simulink model "mrefrobotarm_previous_y_previous_u_previous_ref_cex_3"  (R2018b)
settings: Solver=FixedStepAuto  StartTime=0.0  StopTime=20  RelTol=1e-3  AbsTol=1e-6
undefined symbols (not defined in the file or in its folder): cc, options
libraries: neural x396, simulink x2
(part 5 of 15)

== system mrefrobotarm_previous_y_previous_u_previous_ref_cex_3/cex_m1/Layer 3/Delays 1 ==
  "p{3}" : Inport  PortDimensions=30
      mask Display: e = 0.06;c1 = [120 230 180]/255;c2 = ([120 230 180]+0)/(256+128);c3 = ([120 230 180]+128)/(256+128);patch([0 1 1 0],[0 0 1 1],c1);patch([0 1 1 1-e 1-e 0+e],[0 0 1 1-e 0+e 0+e],c2);patch([0 0 1 1-e 0+e 0+e],[0 1 1 1-e 1-e 0+e],c3);plot([0 1 1 0 0],[0 0 1 1 0]);
  mux : Mux  Inputs=1
      mask Display: e = 0.06;c1 = [120 150 230]/255;c2 = ([120 150 230]+0)/383;c3 = ([120 150 230]+128)/383;patch([0 1 1 0],[0 0 1 1],c1);patch([0 1 1 1-e 1-e 0+e],[0 0 1 1-e 0+e 0+e],c2);patch([0 0 1 1-e 0+e 0+e],[0 1 1 1-e 1-e 0+e],c3);plot([0 1 1 0 0],[0 0 1 1 0]);disp('Mux')
  "pd{3,2}" : Outport
      mask Display: e = 0.06;c1 = [120 230 180]/255;c2 = ([120 230 180]+0)/(256+128);c3 = ([120 230 180]+128)/(256+128);patch([0 1 1 0],[0 0 1 1],c1);patch([0 1 1 1-e 1-e 0+e],[0 0 1 1-e 0+e 0+e],c2);patch([0 0 1 1-e 0+e 0+e],[0 1 1 1-e 1-e 0+e],c3);plot([0 1 1 0 0],[0 0 1 1 0]);
  wires:
  "p{3}"/1 -> mux/1
  mux/1 -> "pd{3,2}"/1

== system mrefrobotarm_previous_y_previous_u_previous_ref_cex_3/cex_m1/Layer 3/LW{3,2} ==
  "ad{3,2}" : Inport  PortDimensions=30
      mask Display: e = 0.06;c1 = [120 230 180]/255;c2 = ([120 230 180]+0)/(256+128);c3 = ([120 230 180]+128)/(256+128);patch([0 1 1 0],[0 0 1 1],c1);patch([0 1 1 1-e 1-e 0+e],[0 0 1 1-e 0+e 0+e],c2);patch([0 0 1 1-e 0+e 0+e],[0 1 1 1-e 1-e 0+e],c3);plot([0 1 1 0 0],[0 0 1 1 0]);
  "IW{3,2}(1,:)'" : Constant  Value=[0.0255900601227965381057050109347983379848301410675048828125;-0.2445332719523497233549136353758512996137142181396484375;0.2132234013283009488315400403735111467540264129638671875;-0.0515001036072283702171858976726070977747440338134765625;-0.19351367720373280345569355631596408784389495849609375;0.376109267327173701911391390240169130265712738037109375;0.0666749128615344577308832185735809616744518280029296875;-0.44077680308893107952172840668936260044574737548828125;-0.1774770708842355604328844265182851813733577728271484375;-0.054251675677824177934649441112924250774085521697998046875;0.407756480058180159620206950421561487019062042236328125;-0.11043832971419904886989371561867301352322101593017578125;-0.06656652324338363513334115850739181041717529296875;-0.309772314576237606242870015194057486951351165771484375;-0.2782579958208721837564780798857100307941436767578125;0.0014079282704737897634339471863995640887878835201263427734375;0.164750395979450681149813817683025263249874114990234375;0.03374371873575258973243506943617830984294414520263671875;-0.11697430223199604959471997744913096539676189422607421875;-0.377976875689660485324594674239051528275012969970703125;0.180234815360957700836053163584438152611255645751953125;0.049494338029175431736828016937579377554357051849365234375;-0.541724329864333054018743496271781623363494873046875;0.70957921545389057715880198884406127035617828369140625;-0.2236538006543592749242321815472678281366825103759765625;-0.0168625825253284934712727505257134907878935337066650390625;-0.061157151815638820246956441906149848364293575286865234375;0.0962999458349639014809184800469665788114070892333984375;-0.195422183072548050208894210300059057772159576416015625;0.469008564925858462135721538288635201752185821533203125]
      mask Display: e = 0.06;c1 = [120 150 230]/255;c2 = ([120 150 230]+0)/383;c3 = ([120 150 230]+128)/383;patch([0 1 1 0],[0 0 1 1],c1);patch([0 1 1 1-e 1-e 0+e],[0 0 1 1-e 0+e 0+e],c2);patch([0 0 1 1-e 0+e 0+e],[0 1 1 1-e 1-e 0+e],c3);plot([0 1 1 0 0],[0 0 1 1 0]);disp('weights');
  Mux : Mux  Inputs=1
      mask Display: e = 0.06;c1 = [120 150 230]/255;c2 = ([120 150 230]+0)/383;c3 = ([120 150 230]+128)/383;patch([0 1 1 0],[0 0 1 1],c1);patch([0 1 1 1-e 1-e 0+e],[0 0 1 1-e 0+e 0+e],c2);patch([0 0 1 1-e 0+e 0+e],[0 1 1 1-e 1-e 0+e],c3);plot([0 1 1 0 0],[0 0 1 1 0]);disp('Mux');
  dotprod1 : neural/Weight Functions/dotprod
  "lz{3,2}" : Outport
      mask Display: e = 0.06;c1 = [120 230 180]/255;c2 = ([120 230 180]+0)/(256+128);c3 = ([120 230 180]+128)/(256+128);patch([0 1 1 0],[0 0 1 1],c1);patch([0 1 1 1-e 1-e 0+e],[0 0 1 1-e 0+e 0+e],c2);patch([0 0 1 1-e 0+e 0+e],[0 1 1 1-e 1-e 0+e],c3);plot([0 1 1 0 0],[0 0 1 1 0]);
  wires:
  "IW{3,2}(1,:)'"/1 -> dotprod1/1
  "ad{3,2}"/1 -> dotprod1/2
  dotprod1/1 -> Mux/1
  Mux/1 -> "lz{3,2}"/1

== system mrefrobotarm_previous_y_previous_u_previous_ref_cex_3/cex_m2_adapt/Layer 1/Delays 1 ==
  "p{1}" : Inport  PortDimensions=10
      mask Display: e = 0.06;c1 = [120 230 180]/255;c2 = ([120 230 180]+0)/(256+128);c3 = ([120 230 180]+128)/(256+128);patch([0 1 1 0],[0 0 1 1],c1);patch([0 1 1 1-e 1-e 0+e],[0 0 1 1-e 0+e 0+e],c2);patch([0 0 1 1-e 0+e 0+e],[0 1 1 1-e 1-e 0+e],c3);plot([0 1 1 0 0],[0 0 1 1 0]);
  mux : Mux  Inputs=1
      mask Display: e = 0.06;c1 = [120 150 230]/255;c2 = ([120 150 230]+0)/383;c3 = ([120 150 230]+128)/383;patch([0 1 1 0],[0 0 1 1],c1);patch([0 1 1 1-e 1-e 0+e],[0 0 1 1-e 0+e 0+e],c2);patch([0 0 1 1-e 0+e 0+e],[0 1 1 1-e 1-e 0+e],c3);plot([0 1 1 0 0],[0 0 1 1 0]);disp('Mux')
  "pd{1,1}" : Outport
      mask Display: e = 0.06;c1 = [120 230 180]/255;c2 = ([120 230 180]+0)/(256+128);c3 = ([120 230 180]+128)/(256+128);patch([0 1 1 0],[0 0 1 1],c1);patch([0 1 1 1-e 1-e 0+e],[0 0 1 1-e 0+e 0+e],c2);patch([0 0 1 1-e 0+e 0+e],[0 1 1 1-e 1-e 0+e],c3);plot([0 1 1 0 0],[0 0 1 1 0]);
  wires:
  "p{1}"/1 -> mux/1
  mux/1 -> "pd{1,1}"/1

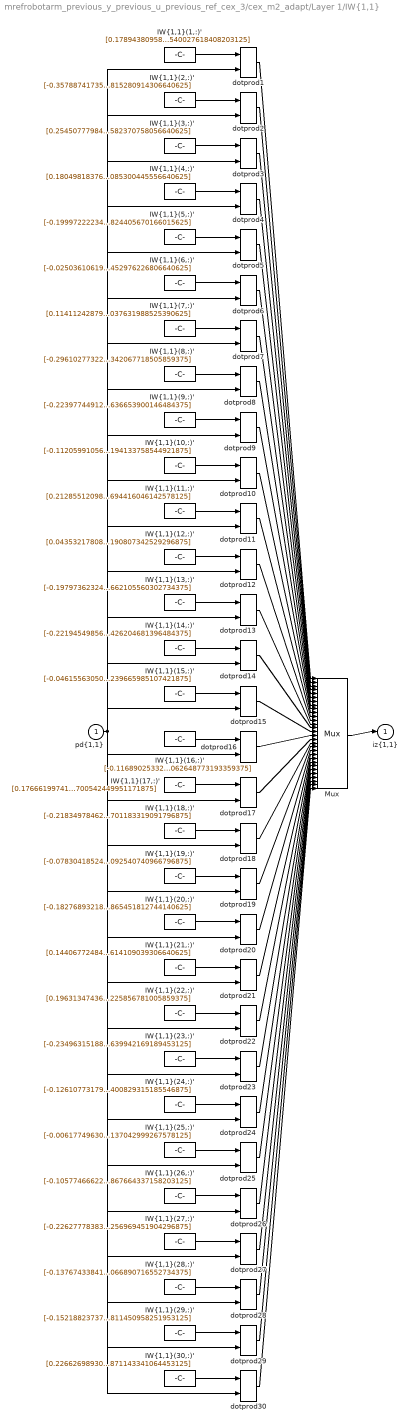
== system mrefrobotarm_previous_y_previous_u_previous_ref_cex_3/cex_m2_adapt/Layer 1/IW{1,1} ==
  "pd{1,1}" : Inport  PortDimensions=10
      mask Display: e = 0.06;c1 = [120 230 180]/255;c2 = ([120 230 180]+0)/(256+128);c3 = ([120 230 180]+128)/(256+128);patch([0 1 1 0],[0 0 1 1],c1);patch([0 1 1 1-e 1-e 0+e],[0 0 1 1-e 0+e 0+e],c2);patch([0 0 1 1-e 0+e 0+e],[0 1 1 1-e 1-e 0+e],c3);plot([0 1 1 0 0],[0 0 1 1 0]);
  "IW{1,1}(1,:)'" : Constant  Value=[0.17894380958113875745851828469312749803066253662109375;0.0268071317300851152953811151746776886284351348876953125;-0.0194245512122687945255616881468085921369493007659912109375;-0.08160327981400332386652252125713857822120189666748046875;-0.09141169433945516009654141953433281742036342620849609375;-0.0300313493066236281148206899160868488252162933349609375;-0.282419827211167984160056221298873424530029296875;0.1311114560309999121923141274237423203885555267333984375;-0.18958968204741710739114068928756751120090484619140625;0.2425038701812252117662183081847615540027618408203125]
      mask Display: e = 0.06;c1 = [120 150 230]/255;c2 = ([120 150 230]+0)/383;c3 = ([120 150 230]+128)/383;patch([0 1 1 0],[0 0 1 1],c1);patch([0 1 1 1-e 1-e 0+e],[0 0 1 1-e 0+e 0+e],c2);patch([0 0 1 1-e 0+e 0+e],[0 1 1 1-e 1-e 0+e],c3);plot([0 1 1 0 0],[0 0 1 1 0]);disp('Weights');
  "IW{1,1}(10,:)'" : Constant  Value=[-0.11205991056579979459062457181062200106680393218994140625;0.357141388765579048669707162844133563339710235595703125;-0.24716782224828592884335876078694127500057220458984375;0.0269643266049996131739074911592979333363473415374755859375;0.33336725590618654369023943218053318560123443603515625;-0.3923495977236670650967198525904677808284759521484375;0.1045060443543400496846373926018713973462581634521484375;-0.06697855843020487920380645618934067897498607635498046875;-0.0864082527450108772715253735441365279257297515869140625;-0.39109248089432480099958411301486194133758544921875]
      mask Display: e = 0.06;c1 = [120 150 230]/255;c2 = ([120 150 230]+0)/383;c3 = ([120 150 230]+128)/383;patch([0 1 1 0],[0 0 1 1],c1);patch([0 1 1 1-e 1-e 0+e],[0 0 1 1-e 0+e 0+e],c2);patch([0 0 1 1-e 0+e 0+e],[0 1 1 1-e 1-e 0+e],c3);plot([0 1 1 0 0],[0 0 1 1 0]);disp('Weights');
  "IW{1,1}(11,:)'" : Constant  Value=[0.2128551209829567525400051408723811618983745574951171875;-0.2022275282815631236577047502578352577984333038330078125;0.0248801394003134446197833540281862951815128326416015625;-0.152377187466551433647765634304960258305072784423828125;0.01342328889111928623412151040383832878433167934417724609375;0.33377738714321558699538172731990925967693328857421875;-0.12204906903726205069649068946091574616730213165283203125;0.154449232987741658096325636506662704050540924072265625;-0.029966565392852896609898749602507450617849826812744140625;0.1513983111497898825792418620039825327694416046142578125]
      mask Display: e = 0.06;c1 = [120 150 230]/255;c2 = ([120 150 230]+0)/383;c3 = ([120 150 230]+128)/383;patch([0 1 1 0],[0 0 1 1],c1);patch([0 1 1 1-e 1-e 0+e],[0 0 1 1-e 0+e 0+e],c2);patch([0 0 1 1-e 0+e 0+e],[0 1 1 1-e 1-e 0+e],c3);plot([0 1 1 0 0],[0 0 1 1 0]);disp('Weights');
  "IW{1,1}(12,:)'" : Constant  Value=[0.043532178080436627343186017924381303600966930389404296875;-0.41453145188763296236089672675007022917270660400390625;0.215272607105115143522056087022065185010433197021484375;0.1665664633557482066095190020860172808170318603515625;-0.02357860495869094907828156237883376888930797576904296875;0.0857323194401150845411763157244422473013401031494140625;-0.1958108534085869489871356563526205718517303466796875;-0.1625029873389834123020847300722380168735980987548828125;0.25121695445630820575644293057848699390888214111328125;-0.106927667380184832079947909733164124190807342529296875]
      mask Display: e = 0.06;c1 = [120 150 230]/255;c2 = ([120 150 230]+0)/383;c3 = ([120 150 230]+128)/383;patch([0 1 1 0],[0 0 1 1],c1);patch([0 1 1 1-e 1-e 0+e],[0 0 1 1-e 0+e 0+e],c2);patch([0 0 1 1-e 0+e 0+e],[0 1 1 1-e 1-e 0+e],c3);plot([0 1 1 0 0],[0 0 1 1 0]);disp('Weights');
  "IW{1,1}(13,:)'" : Constant  Value=[-0.197973623241752105794688532114378176629543304443359375;0.1845413812524343832865980630231206305325031280517578125;-0.06383679347059974251710201542664435692131519317626953125;0.2121214746879949430979905855565448291599750518798828125;-0.1380893753585880900924820480213384144008159637451171875;0.038970623662596674818825448483039508573710918426513671875;0.1056184031157495761821252244772040285170078277587890625;-0.1502218965172570086519243659495259635150432586669921875;-0.246327164138165410900427332308026961982250213623046875;0.2171770133514413225750416813752963207662105560302734375]
      mask Display: e = 0.06;c1 = [120 150 230]/255;c2 = ([120 150 230]+0)/383;c3 = ([120 150 230]+128)/383;patch([0 1 1 0],[0 0 1 1],c1);patch([0 1 1 1-e 1-e 0+e],[0 0 1 1-e 0+e 0+e],c2);patch([0 0 1 1-e 0+e 0+e],[0 1 1 1-e 1-e 0+e],c3);plot([0 1 1 0 0],[0 0 1 1 0]);disp('Weights');
  "IW{1,1}(14,:)'" : Constant  Value=[-0.2219454985619064846247283639968372881412506103515625;-0.031461568819169304089822247760821483097970485687255859375;0.25100732039812767570907681147218681871891021728515625;-0.071675964588810925359751990981749258935451507568359375;-0.017276940888944262997295453487822669558227062225341796875;0.18731594061744616386278039499302394688129425048828125;0.190073867922183448175843523131334222853183746337890625;0.25628758967802023338578010225319303572177886962890625;-0.12311552773296086105148106071283109486103057861328125;0.0836877380832282413702927215126692317426204681396484375]
      mask Display: e = 0.06;c1 = [120 150 230]/255;c2 = ([120 150 230]+0)/383;c3 = ([120 150 230]+128)/383;patch([0 1 1 0],[0 0 1 1],c1);patch([0 1 1 1-e 1-e 0+e],[0 0 1 1-e 0+e 0+e],c2);patch([0 0 1 1-e 0+e 0+e],[0 1 1 1-e 1-e 0+e],c3);plot([0 1 1 0 0],[0 0 1 1 0]);disp('Weights');
  "IW{1,1}(15,:)'" : Constant  Value=[-0.0461556305026336877173065431634313426911830902099609375;-0.150134721130089798801776623804471455514430999755859375;0.009230602670664188325044818839160143397748470306396484375;-0.263036107154839104982357866902020759880542755126953125;-0.23279760428147711071034109409083612263202667236328125;-0.2026113135926179975587757553512346930801868438720703125;0.051737200499545492327069240445780451409518718719482421875;-0.209756927138399051901984648793586529791355133056640625;0.18107018174338918026222700063954107463359832763671875;-0.037977675462847075571470867316747899167239665985107421875]
      mask Display: e = 0.06;c1 = [120 150 230]/255;c2 = ([120 150 230]+0)/383;c3 = ([120 150 230]+128)/383;patch([0 1 1 0],[0 0 1 1],c1);patch([0 1 1 1-e 1-e 0+e],[0 0 1 1-e 0+e 0+e],c2);patch([0 0 1 1-e 0+e 0+e],[0 1 1 1-e 1-e 0+e],c3);plot([0 1 1 0 0],[0 0 1 1 0]);disp('Weights');
  "IW{1,1}(16,:)'" : Constant  Value=[-0.116890253323373605187640578151331283152103424072265625;0.1948278121702989029717656421780702657997608184814453125;0.2451443399859792038331107733029057271778583526611328125;0.0631447386421812861811986294924281537532806396484375;-0.17107126514984816179065774122136645019054412841796875;0.2286361380735318082901841307830181904137134552001953125;0.1679551899195639574902116919474792666733264923095703125;-0.1360221986945425454162972300764522515237331390380859375;0.1710850103284725365337948232991038821637630462646484375;-0.03517712954871109187759969927355996333062648773193359375]
      mask Display: e = 0.06;c1 = [120 150 230]/255;c2 = ([120 150 230]+0)/383;c3 = ([120 150 230]+128)/383;patch([0 1 1 0],[0 0 1 1],c1);patch([0 1 1 1-e 1-e 0+e],[0 0 1 1-e 0+e 0+e],c2);patch([0 0 1 1-e 0+e 0+e],[0 1 1 1-e 1-e 0+e],c3);plot([0 1 1 0 0],[0 0 1 1 0]);disp('Weights');
  "IW{1,1}(17,:)'" : Constant  Value=[0.1766619974178879892701132803267682902514934539794921875;-0.0792409472181059559847682294275728054344654083251953125;-0.0793088341233295912591216847431496717035770416259765625;-0.1959233532531541588372903106574085541069507598876953125;0.11565209295813162759802850132473395206034183502197265625;0.00787878799489242533093946718736333423294126987457275390625;0.042692546684134226320228577833404415287077426910400390625;-0.209397876134871430142680992503301240503787994384765625;-0.17372430623133772176203137860284186899662017822265625;-0.30776366573309743568387375489692203700542449951171875]
      mask Display: e = 0.06;c1 = [120 150 230]/255;c2 = ([120 150 230]+0)/383;c3 = ([120 150 230]+128)/383;patch([0 1 1 0],[0 0 1 1],c1);patch([0 1 1 1-e 1-e 0+e],[0 0 1 1-e 0+e 0+e],c2);patch([0 0 1 1-e 0+e 0+e],[0 1 1 1-e 1-e 0+e],c3);plot([0 1 1 0 0],[0 0 1 1 0]);disp('Weights');
  "IW{1,1}(18,:)'" : Constant  Value=[-0.218349784629069620933705664356239140033721923828125;0.0642278208810374284798427879650262184441089630126953125;-0.0619524210695374388802036946799489669501781463623046875;0.09804765153544270361862800200469791889190673828125;-0.1940721708608581508315182873047888278961181640625;0.10055382144939296884533774800729588605463504791259765625;0.055125079744373917112199023904395289719104766845703125;-0.22257044783044499514090830416535027325153350830078125;0.307695206730231929359575815396965481340885162353515625;0.035102723566185704828779279296213644556701183319091796875]
      mask Display: e = 0.06;c1 = [120 150 230]/255;c2 = ([120 150 230]+0)/383;c3 = ([120 150 230]+128)/383;patch([0 1 1 0],[0 0 1 1],c1);patch([0 1 1 1-e 1-e 0+e],[0 0 1 1-e 0+e 0+e],c2);patch([0 0 1 1-e 0+e 0+e],[0 1 1 1-e 1-e 0+e],c3);plot([0 1 1 0 0],[0 0 1 1 0]);disp('Weights');
  "IW{1,1}(19,:)'" : Constant  Value=[-0.0783041852438026986238384097305242903530597686767578125;-0.110159278051770892492555731223546899855136871337890625;0.0703702840684951869132390811500954441726207733154296875;-0.07371581746469789420128648771424195729196071624755859375;0.249837105675603743382140464746044017374515533447265625;-0.1447885961919746222736904428529669530689716339111328125;0.321300374598912752421853156192810274660587310791015625;0.0142112607252117585654449527510223560966551303863525390625;-0.2097588763900186392685753844489227049052715301513671875;-0.137897701114751913831213414596277289092540740966796875]
      mask Display: e = 0.06;c1 = [120 150 230]/255;c2 = ([120 150 230]+0)/383;c3 = ([120 150 230]+128)/383;patch([0 1 1 0],[0 0 1 1],c1);patch([0 1 1 1-e 1-e 0+e],[0 0 1 1-e 0+e 0+e],c2);patch([0 0 1 1-e 0+e 0+e],[0 1 1 1-e 1-e 0+e],c3);plot([0 1 1 0 0],[0 0 1 1 0]);disp('Weights');
  "IW{1,1}(2,:)'" : Constant  Value=[-0.3578874173535078195840242187841795384883880615234375;-0.170151089097431207353139370752614922821521759033203125;0.1283993877341979839012964248468051664531230926513671875;0.0278821277396804866055557425852384767495095729827880859375;0.241336606408127651857142836888669990003108978271484375;-0.088299581297500984167214710396365262567996978759765625;-0.05964540699157604153324285789494751952588558197021484375;-0.18177101439334253374369154698797501623630523681640625;-0.202751370739727987402289954843581654131412506103515625;0.03612164991689260917784309867784031666815280914306640625]
      mask Display: e = 0.06;c1 = [120 150 230]/255;c2 = ([120 150 230]+0)/383;c3 = ([120 150 230]+128)/383;patch([0 1 1 0],[0 0 1 1],c1);patch([0 1 1 1-e 1-e 0+e],[0 0 1 1-e 0+e 0+e],c2);patch([0 0 1 1-e 0+e 0+e],[0 1 1 1-e 1-e 0+e],c3);plot([0 1 1 0 0],[0 0 1 1 0]);disp('Weights');
  "IW{1,1}(20,:)'" : Constant  Value=[-0.182768932186715804544263619391131214797496795654296875;0.429775783628007890246891520291683264076709747314453125;0.047518314508741339718955742910111439414322376251220703125;-0.051709077215492692258802520655081025324761867523193359375;0.091944243252948643085886715198284946382045745849609375;-0.378830904703480075834676199519890360534191131591796875;-0.03264809407481177039311859289227868430316448211669921875;-0.035928795977489068336208077880655764602124691009521484375;-0.0821954152999051779193706579462741501629352569580078125;-0.122911018759520873633306337069370783865451812744140625]
      mask Display: e = 0.06;c1 = [120 150 230]/255;c2 = ([120 150 230]+0)/383;c3 = ([120 150 230]+128)/383;patch([0 1 1 0],[0 0 1 1],c1);patch([0 1 1 1-e 1-e 0+e],[0 0 1 1-e 0+e 0+e],c2);patch([0 0 1 1-e 0+e 0+e],[0 1 1 1-e 1-e 0+e],c3);plot([0 1 1 0 0],[0 0 1 1 0]);disp('Weights');
  "IW{1,1}(21,:)'" : Constant  Value=[0.1440677248405341226433762358283274807035923004150390625;0.05674263640774103445441056692288839258253574371337890625;0.186993057845454779819505120030953548848628997802734375;-0.1647920441410975767038138428688398562371730804443359375;-0.23737996741754530116708110654144547879695892333984375;0.253688660892035511285058646535617299377918243408203125;-0.2346548398854706451999163618893362581729888916015625;0.0215902337998425848664130199949795496650040149688720703125;0.2383889116336310731725234290934167802333831787109375;-0.0025995181104539661666452676769267782219685614109039306640625]
      mask Display: e = 0.06;c1 = [120 150 230]/255;c2 = ([120 150 230]+0)/383;c3 = ([120 150 230]+128)/383;patch([0 1 1 0],[0 0 1 1],c1);patch([0 1 1 1-e 1-e 0+e],[0 0 1 1-e 0+e 0+e],c2);patch([0 0 1 1-e 0+e 0+e],[0 1 1 1-e 1-e 0+e],c3);plot([0 1 1 0 0],[0 0 1 1 0]);disp('Weights');
  "IW{1,1}(22,:)'" : Constant  Value=[0.1963134743628309752949689936940558254718780517578125;-0.05200275022295146321038572523320908658206462860107421875;-0.2715367927651737289806987973861396312713623046875;-0.08952620051789726696167548425364657305181026458740234375;-0.036953019016694517440146938724865322001278400421142578125;0.004476533827437712519115020626259138225577771663665771484375;0.259201846168678973203469695363310165703296661376953125;-0.08894573404800827642890936886033159680664539337158203125;0.032269069594959988445115328659085207618772983551025390625;0.306951271732894992450013660345575772225856781005859375]
      mask Display: e = 0.06;c1 = [120 150 230]/255;c2 = ([120 150 230]+0)/383;c3 = ([120 150 230]+128)/383;patch([0 1 1 0],[0 0 1 1],c1);patch([0 1 1 1-e 1-e 0+e],[0 0 1 1-e 0+e 0+e],c2);patch([0 0 1 1-e 0+e 0+e],[0 1 1 1-e 1-e 0+e],c3);plot([0 1 1 0 0],[0 0 1 1 0]);disp('Weights');
  "IW{1,1}(23,:)'" : Constant  Value=[-0.2349631518819057240943237729879911057651042938232421875;-0.17641433096250180856401357232243753969669342041015625;0.23491215286060407319013165761134587228298187255859375;0.0979759738956398062992292352646472863852977752685546875;0.275412544487549648675184243984404020011425018310546875;-0.006673035133562527261574803816301937331445515155792236328125;-0.086308845438423376084102756067295558750629425048828125;-0.04925444461655315020465195630094967782497406005859375;0.311981159375483707574261416084482334554195404052734375;-0.13017093754148068018849926374969072639942169189453125]
      mask Display: e = 0.06;c1 = [120 150 230]/255;c2 = ([120 150 230]+0)/383;c3 = ([120 150 230]+128)/383;patch([0 1 1 0],[0 0 1 1],c1);patch([0 1 1 1-e 1-e 0+e],[0 0 1 1-e 0+e 0+e],c2);patch([0 0 1 1-e 0+e 0+e],[0 1 1 1-e 1-e 0+e],c3);plot([0 1 1 0 0],[0 0 1 1 0]);disp('Weights');
  "IW{1,1}(24,:)'" : Constant  Value=[-0.126107731797233502124555570844677276909351348876953125;0.0845353935998513772442919389504822902381420135498046875;-0.170961691516502922727482882692129351198673248291015625;0.2911848648253305693600623271777294576168060302734375;0.1152242375241279426223428572484408505260944366455078125;0.270250526997318607502762688454822637140750885009765625;0.11501804092393873302224704957552603445947170257568359375;0.06893195638638706379541787327980273403227329254150390625;0.09231210104422175877214584716057288460433483123779296875;0.12574616199281507533669355325400829315185546875]
      mask Display: e = 0.06;c1 = [120 150 230]/255;c2 = ([120 150 230]+0)/383;c3 = ([120 150 230]+128)/383;patch([0 1 1 0],[0 0 1 1],c1);patch([0 1 1 1-e 1-e 0+e],[0 0 1 1-e 0+e 0+e],c2);patch([0 0 1 1-e 0+e 0+e],[0 1 1 1-e 1-e 0+e],c3);plot([0 1 1 0 0],[0 0 1 1 0]);disp('Weights');
  "IW{1,1}(25,:)'" : Constant  Value=[-0.0061774963028770855932858552250763750635087490081787109375;0.1585491037024161775637054461185471154749393463134765625;0.188599532141205228352731637642136774957180023193359375;-0.01688017055565992075027992314062430523335933685302734375;-0.18879192571435854386407982019591145217418670654296875;0.1272448344067560188630494621975230984389781951904296875;-0.018569046672616905391262065450064255855977535247802734375;0.2719719856826794401882807505899108946323394775390625;0.11406227701772338190000510849131387658417224884033203125;-0.2380939274560498752908443975684349425137042999267578125]
      mask Display: e = 0.06;c1 = [120 150 230]/255;c2 = ([120 150 230]+0)/383;c3 = ([120 150 230]+128)/383;patch([0 1 1 0],[0 0 1 1],c1);patch([0 1 1 1-e 1-e 0+e],[0 0 1 1-e 0+e 0+e],c2);patch([0 0 1 1-e 0+e 0+e],[0 1 1 1-e 1-e 0+e],c3);plot([0 1 1 0 0],[0 0 1 1 0]);disp('Weights');
  "IW{1,1}(26,:)'" : Constant  Value=[-0.10577466622952902408627551267272792756557464599609375;0.178203524722881312403188758253236301243305206298828125;-0.257770785536782287561408111287164501845836639404296875;-0.12118946165142341353515575974597595632076263427734375;0.1079912289210649134485464628596673719584941864013671875;0.03241305524148041516951934681856073439121246337890625;0.23392595501652213574317329403129406273365020751953125;0.04862524796426924422743098830324015580117702484130859375;-0.07777126056271836673783326432385365478694438934326171875;-0.066068618504620257869675015172106213867664337158203125]
      mask Display: e = 0.06;c1 = [120 150 230]/255;c2 = ([120 150 230]+0)/383;c3 = ([120 150 230]+128)/383;patch([0 1 1 0],[0 0 1 1],c1);patch([0 1 1 1-e 1-e 0+e],[0 0 1 1-e 0+e 0+e],c2);patch([0 0 1 1-e 0+e 0+e],[0 1 1 1-e 1-e 0+e],c3);plot([0 1 1 0 0],[0 0 1 1 0]);disp('Weights');
  "IW{1,1}(27,:)'" : Constant  Value=[-0.22627778383142194140731362494989298284053802490234375;0.2283804303486903497510951410731649957597255706787109375;-0.04633207616607355749938079725325223989784717559814453125;-0.2155678259000181895554959510263870470225811004638671875;-0.024473322781653643331889469436646322719752788543701171875;-0.061312110441402466187721387314013554714620113372802734375;0.192636598116036783512328156575676985085010528564453125;0.2137994347702246444864471186519949696958065032958984375;0.240218978868222909905938422525650821626186370849609375;0.00468413039874411400720344289538843440823256969451904296875]
      mask Display: e = 0.06;c1 = [120 150 230]/255;c2 = ([120 150 230]+0)/383;c3 = ([120 150 230]+128)/383;patch([0 1 1 0],[0 0 1 1],c1);patch([0 1 1 1-e 1-e 0+e],[0 0 1 1-e 0+e 0+e],c2);patch([0 0 1 1-e 0+e 0+e],[0 1 1 1-e 1-e 0+e],c3);plot([0 1 1 0 0],[0 0 1 1 0]);disp('Weights');
  "IW{1,1}(28,:)'" : Constant  Value=[-0.1376743384100590217311577134751132689416408538818359375;0.135728354626229730239828086268971674144268035888671875;0.109024380491910488633067188857239671051502227783203125;-0.020932506514744549097617465349685517139732837677001953125;0.1596172013299924363760595724670565687119960784912109375;-0.2246346884976990754267944794264622032642364501953125;-0.126744927810719054672716765708173625171184539794921875;0.152022505625554471553328994559706188738346099853515625;0.2181400746204700258346065311343409121036529541015625;-0.047226325411993307079594472952521755360066890716552734375]
      mask Display: e = 0.06;c1 = [120 150 230]/255;c2 = ([120 150 230]+0)/383;c3 = ([120 150 230]+128)/383;patch([0 1 1 0],[0 0 1 1],c1);patch([0 1 1 1-e 1-e 0+e],[0 0 1 1-e 0+e 0+e],c2);patch([0 0 1 1-e 0+e 0+e],[0 1 1 1-e 1-e 0+e],c3);plot([0 1 1 0 0],[0 0 1 1 0]);disp('Weights');
  "IW{1,1}(29,:)'" : Constant  Value=[-0.1521882373734292637212917043143534101545810699462890625;-0.0458248690782084022732334460670244880020618438720703125;0.07555221417059405919491865688542020507156848907470703125;-0.1852621927616607544475613167378469370305538177490234375;0.15125110154184862043535986231290735304355621337890625;-0.1412090535903816890250794813255197368562221527099609375;-0.08681811528340076244969480967483832500874996185302734375;-0.224873363801992687260877801236347295343875885009765625;-0.165199621824701325945028429487138055264949798583984375;0.157553748575570029544223871198482811450958251953125]
      mask Display: e = 0.06;c1 = [120 150 230]/255;c2 = ([120 150 230]+0)/383;c3 = ([120 150 230]+128)/383;patch([0 1 1 0],[0 0 1 1],c1);patch([0 1 1 1-e 1-e 0+e],[0 0 1 1-e 0+e 0+e],c2);patch([0 0 1 1-e 0+e 0+e],[0 1 1 1-e 1-e 0+e],c3);plot([0 1 1 0 0],[0 0 1 1 0]);disp('Weights');
  "IW{1,1}(3,:)'" : Constant  Value=[0.2545077798497317189685418270528316497802734375;0.040200776831324842863768509459987399168312549591064453125;0.16885528047504616555585243986570276319980621337890625;0.227543951883704076433190266470774076879024505615234375;0.2384163836713796558175459949779906310141086578369140625;0.1413290689938786204304932425657170824706554412841796875;0.10575857589675634329307030156996916048228740692138671875;0.133407682047404663183698403372545726597309112548828125;0.12030518109430683726390753918167320080101490020751953125;0.11598616257945094931702811891227611340582370758056640625]
      mask Display: e = 0.06;c1 = [120 150 230]/255;c2 = ([120 150 230]+0)/383;c3 = ([120 150 230]+128)/383;patch([0 1 1 0],[0 0 1 1],c1);patch([0 1 1 1-e 1-e 0+e],[0 0 1 1-e 0+e 0+e],c2);patch([0 0 1 1-e 0+e 0+e],[0 1 1 1-e 1-e 0+e],c3);plot([0 1 1 0 0],[0 0 1 1 0]);disp('Weights');
  "IW{1,1}(30,:)'" : Constant  Value=[0.226626989308528814515142357777222059667110443115234375;0.1400904348982205671614309494543704204261302947998046875;-0.11186941054087540248218601846019737422466278076171875;0.2012528084778613945982073119012056849896907806396484375;-0.018626897424557094240515908722954918630421161651611328125;-0.200639757261653117748068098080693744122982025146484375;-0.0961578448371694094465311763997306115925312042236328125;-0.177214676264387749338169442125945352017879486083984375;0.031918329000240552861811238472000695765018463134765625;0.266965554029287677195725336787290871143341064453125]
      mask Display: e = 0.06;c1 = [120 150 230]/255;c2 = ([120 150 230]+0)/383;c3 = ([120 150 230]+128)/383;patch([0 1 1 0],[0 0 1 1],c1);patch([0 1 1 1-e 1-e 0+e],[0 0 1 1-e 0+e 0+e],c2);patch([0 0 1 1-e 0+e 0+e],[0 1 1 1-e 1-e 0+e],c3);plot([0 1 1 0 0],[0 0 1 1 0]);disp('Weights');
  "IW{1,1}(4,:)'" : Constant  Value=[0.180498183761611807884861491402261890470981597900390625;-0.2288560682142836977259747754942509345710277557373046875;0.181865366464034339255562144899158738553524017333984375;-0.03794964346253447418089166376375942490994930267333984375;-0.00539640154973875484090140020043691038154065608978271484375;0.1827887046756515310175217337018693797290325164794921875;-0.05529857869917853552266251426772214472293853759765625;-0.1474419509970783248586911895472439937293529510498046875;-0.27933067356285434801321798659046180546283721923828125;0.1322504052913414940295666610836633481085300445556640625]
      mask Display: e = 0.06;c1 = [120 150 230]/255;c2 = ([120 150 230]+0)/383;c3 = ([120 150 230]+128)/383;patch([0 1 1 0],[0 0 1 1],c1);patch([0 1 1 1-e 1-e 0+e],[0 0 1 1-e 0+e 0+e],c2);patch([0 0 1 1-e 0+e 0+e],[0 1 1 1-e 1-e 0+e],c3);plot([0 1 1 0 0],[0 0 1 1 0]);disp('Weights');
  "IW{1,1}(5,:)'" : Constant  Value=[-0.199972222347502948114339460516930557787418365478515625;-0.1629616266957280845684152836838620714843273162841796875;-0.1088061844054873106291125850475509651005268096923828125;0.0511308765597847936223985243486822582781314849853515625;-0.0237228601571770163214392113104622694663703441619873046875;0.05171937119826557072155281957748229615390300750732421875;-0.1720231930632351302623561650761985220015048980712890625;-0.2044816792317828146874347794437198899686336517333984375;0.1663037605507071692301224175025708973407745361328125;-0.1391865350676850798805617159814573824405670166015625]
      mask Display: e = 0.06;c1 = [120 150 230]/255;c2 = ([120 150 230]+0)/383;c3 = ([120 150 230]+128)/383;patch([0 1 1 0],[0 0 1 1],c1);patch([0 1 1 1-e 1-e 0+e],[0 0 1 1-e 0+e 0+e],c2);patch([0 0 1 1-e 0+e 0+e],[0 1 1 1-e 1-e 0+e],c3);plot([0 1 1 0 0],[0 0 1 1 0]);disp('Weights');
  "IW{1,1}(6,:)'" : Constant  Value=[-0.025036106197230699466071968117830692790448665618896484375;-0.004459099454261481083883200682294045691378414630889892578125;0.06640331129765809914378138500978820957243442535400390625;-0.213060680378278355373566910202498547732830047607421875;0.1292960241831762335795730223253485746681690216064453125;-0.134777908717993444298599570174701511859893798828125;-0.2359873783413052594770675796098657883703708648681640625;-0.06528979964846935712952102903727791272103786468505859375;-0.14430156278261174751520456993603147566318511962890625;0.0887677052430439206265333496048697270452976226806640625]
      mask Display: e = 0.06;c1 = [120 150 230]/255;c2 = ([120 150 230]+0)/383;c3 = ([120 150 230]+128)/383;patch([0 1 1 0],[0 0 1 1],c1);patch([0 1 1 1-e 1-e 0+e],[0 0 1 1-e 0+e 0+e],c2);patch([0 0 1 1-e 0+e 0+e],[0 1 1 1-e 1-e 0+e],c3);plot([0 1 1 0 0],[0 0 1 1 0]);disp('Weights');
  "IW{1,1}(7,:)'" : Constant  Value=[0.11411242879864545718415769215425825677812099456787109375;-0.0719764546582311870448478430262184701859951019287109375;0.2194207952041006548515866825255216099321842193603515625;0.208720306017479206861509055670467205345630645751953125;0.042791162240613418721313365722380694933235645294189453125;0.0121936122546550916589946922385934158228337764739990234375;0.10314935925821260009893620690490934066474437713623046875;0.2155964619388381631193141174662741832435131072998046875;-0.112014458972907127165541396607295610010623931884765625;0.26768961478474262438709274647408165037631988525390625]
      mask Display: e = 0.06;c1 = [120 150 230]/255;c2 = ([120 150 230]+0)/383;c3 = ([120 150 230]+128)/383;patch([0 1 1 0],[0 0 1 1],c1);patch([0 1 1 1-e 1-e 0+e],[0 0 1 1-e 0+e 0+e],c2);patch([0 0 1 1-e 0+e 0+e],[0 1 1 1-e 1-e 0+e],c3);plot([0 1 1 0 0],[0 0 1 1 0]);disp('Weights');
  "IW{1,1}(8,:)'" : Constant  Value=[-0.2961027732226113595714878101716749370098114013671875;-0.07463399570507878166836235322989523410797119140625;-0.23855500073995183907271666612359695136547088623046875;-0.2056116722217617709400627745708334259688854217529296875;0.052565443905320197170993878899025730788707733154296875;-0.1454334110053014939012427930720150470733642578125;0.1567884249944997698822390930217807181179523468017578125;0.1721666479786218284520060706199728883802890777587890625;-0.0903178064951806192084404756315052509307861328125;-0.0525141546112134205426258404258987866342067718505859375]
      mask Display: e = 0.06;c1 = [120 150 230]/255;c2 = ([120 150 230]+0)/383;c3 = ([120 150 230]+128)/383;patch([0 1 1 0],[0 0 1 1],c1);patch([0 1 1 1-e 1-e 0+e],[0 0 1 1-e 0+e 0+e],c2);patch([0 0 1 1-e 0+e 0+e],[0 1 1 1-e 1-e 0+e],c3);plot([0 1 1 0 0],[0 0 1 1 0]);disp('Weights');
  "IW{1,1}(9,:)'" : Constant  Value=[-0.2239774491285566326848055496157030574977397918701171875;-0.1882933671208217030201836905689560808241367340087890625;-0.0257943275412955246028712252837067353539168834686279296875;0.07815168279298902176410734909950406290590763092041015625;0.0356263752072844275264884572607115842401981353759765625;-0.0373208609766592369627602465698146261274814605712890625;-0.28071250177076212395377297070808708667755126953125;0.326090076060244260514053848964977078139781951904296875;0.052075518180411901891790904528534156270325183868408203125;-0.0171626285640969454548976358410072862170636653900146484375]
      mask Display: e = 0.06;c1 = [120 150 230]/255;c2 = ([120 150 230]+0)/383;c3 = ([120 150 230]+128)/383;patch([0 1 1 0],[0 0 1 1],c1);patch([0 1 1 1-e 1-e 0+e],[0 0 1 1-e 0+e 0+e],c2);patch([0 0 1 1-e 0+e 0+e],[0 1 1 1-e 1-e 0+e],c3);plot([0 1 1 0 0],[0 0 1 1 0]);disp('Weights');
  Mux : Mux  Inputs=30
      mask Display: e = 0.06;c1 = [120 150 230]/255;c2 = ([120 150 230]+0)/383;c3 = ([120 150 230]+128)/383;patch([0 1 1 0],[0 0 1 1],c1);patch([0 1 1 1-e 1-e 0+e],[0 0 1 1-e 0+e 0+e],c2);patch([0 0 1 1-e 0+e 0+e],[0 1 1 1-e 1-e 0+e],c3);plot([0 1 1 0 0],[0 0 1 1 0]);disp('Mux');
  dotprod{1..30} (30 alike) : neural/Weight Functions/dotprod
  "iz{1,1}" : Outport
      mask Display: e = 0.06;c1 = [120 230 180]/255;c2 = ([120 230 180]+0)/(256+128);c3 = ([120 230 180]+128)/(256+128);patch([0 1 1 0],[0 0 1 1],c1);patch([0 1 1 1-e 1-e 0+e],[0 0 1 1-e 0+e 0+e],c2);patch([0 0 1 1-e 0+e 0+e],[0 1 1 1-e 1-e 0+e],c3);plot([0 1 1 0 0],[0 0 1 1 0]);
  wires:
  "IW{1,1}(1,:)'"/1 -> dotprod1/1
  "pd{1,1}"/1 -> dotprod1/2, dotprod2/2, dotprod3/2, dotprod4/2, dotprod5/2, dotprod6/2, dotprod7/2, dotprod8/2, dotprod9/2, dotprod10/2, dotprod11/2, dotprod12/2, dotprod13/2, dotprod14/2, dotprod15/2, dotprod16/2, dotprod17/2, dotprod18/2, dotprod19/2, dotprod20/2, dotprod21/2, dotprod22/2, dotprod23/2, dotprod24/2, dotprod25/2, dotprod26/2, dotprod27/2, dotprod28/2, dotprod29/2, dotprod30/2
  dotprod1/1 -> Mux/1
  "IW{1,1}(2,:)'"/1 -> dotprod2/1
  dotprod2/1 -> Mux/2
  "IW{1,1}(3,:)'"/1 -> dotprod3/1
  dotprod3/1 -> Mux/3
  "IW{1,1}(4,:)'"/1 -> dotprod4/1
  dotprod4/1 -> Mux/4
  "IW{1,1}(5,:)'"/1 -> dotprod5/1
  dotprod5/1 -> Mux/5
  "IW{1,1}(6,:)'"/1 -> dotprod6/1
  dotprod6/1 -> Mux/6
  "IW{1,1}(7,:)'"/1 -> dotprod7/1
  dotprod7/1 -> Mux/7
  "IW{1,1}(8,:)'"/1 -> dotprod8/1
  dotprod8/1 -> Mux/8
  "IW{1,1}(9,:)'"/1 -> dotprod9/1
  dotprod9/1 -> Mux/9
  "IW{1,1}(10,:)'"/1 -> dotprod10/1
  dotprod10/1 -> Mux/10
  "IW{1,1}(11,:)'"/1 -> dotprod11/1
  dotprod11/1 -> Mux/11
  "IW{1,1}(12,:)'"/1 -> dotprod12/1
  dotprod12/1 -> Mux/12
  "IW{1,1}(13,:)'"/1 -> dotprod13/1
  dotprod13/1 -> Mux/13
  "IW{1,1}(14,:)'"/1 -> dotprod14/1
  dotprod14/1 -> Mux/14
  "IW{1,1}(15,:)'"/1 -> dotprod15/1
  dotprod15/1 -> Mux/15
  "IW{1,1}(16,:)'"/1 -> dotprod16/1
  dotprod16/1 -> Mux/16
  "IW{1,1}(17,:)'"/1 -> dotprod17/1
  dotprod17/1 -> Mux/17
  "IW{1,1}(18,:)'"/1 -> dotprod18/1
  dotprod18/1 -> Mux/18
  "IW{1,1}(19,:)'"/1 -> dotprod19/1
  dotprod19/1 -> Mux/19
  "IW{1,1}(20,:)'"/1 -> dotprod20/1
  dotprod20/1 -> Mux/20
  "IW{1,1}(21,:)'"/1 -> dotprod21/1
  dotprod21/1 -> Mux/21
  "IW{1,1}(22,:)'"/1 -> dotprod22/1
  dotprod22/1 -> Mux/22
  "IW{1,1}(23,:)'"/1 -> dotprod23/1
  dotprod23/1 -> Mux/23
  "IW{1,1}(24,:)'"/1 -> dotprod24/1
  dotprod24/1 -> Mux/24
  "IW{1,1}(25,:)'"/1 -> dotprod25/1
  dotprod25/1 -> Mux/25
  "IW{1,1}(26,:)'"/1 -> dotprod26/1
  dotprod26/1 -> Mux/26
  "IW{1,1}(27,:)'"/1 -> dotprod27/1
  dotprod27/1 -> Mux/27
  "IW{1,1}(28,:)'"/1 -> dotprod28/1
  dotprod28/1 -> Mux/28
  "IW{1,1}(29,:)'"/1 -> dotprod29/1
  dotprod29/1 -> Mux/29
  "IW{1,1}(30,:)'"/1 -> dotprod30/1
  dotprod30/1 -> Mux/30
  Mux/1 -> "iz{1,1}"/1

== system mrefrobotarm_previous_y_previous_u_previous_ref_cex_3/cex_m2_adapt/Layer 2/Delays 1 ==
  "p{2}" : Inport  PortDimensions=30
      mask Display: e = 0.06;c1 = [120 230 180]/255;c2 = ([120 230 180]+0)/(256+128);c3 = ([120 230 180]+128)/(256+128);patch([0 1 1 0],[0 0 1 1],c1);patch([0 1 1 1-e 1-e 0+e],[0 0 1 1-e 0+e 0+e],c2);patch([0 0 1 1-e 0+e 0+e],[0 1 1 1-e 1-e 0+e],c3);plot([0 1 1 0 0],[0 0 1 1 0]);
  mux : Mux  Inputs=1
      mask Display: e = 0.06;c1 = [120 150 230]/255;c2 = ([120 150 230]+0)/383;c3 = ([120 150 230]+128)/383;patch([0 1 1 0],[0 0 1 1],c1);patch([0 1 1 1-e 1-e 0+e],[0 0 1 1-e 0+e 0+e],c2);patch([0 0 1 1-e 0+e 0+e],[0 1 1 1-e 1-e 0+e],c3);plot([0 1 1 0 0],[0 0 1 1 0]);disp('Mux')
  "pd{2,1}" : Outport
      mask Display: e = 0.06;c1 = [120 230 180]/255;c2 = ([120 230 180]+0)/(256+128);c3 = ([120 230 180]+128)/(256+128);patch([0 1 1 0],[0 0 1 1],c1);patch([0 1 1 1-e 1-e 0+e],[0 0 1 1-e 0+e 0+e],c2);patch([0 0 1 1-e 0+e 0+e],[0 1 1 1-e 1-e 0+e],c3);plot([0 1 1 0 0],[0 0 1 1 0]);
  wires:
  "p{2}"/1 -> mux/1
  mux/1 -> "pd{2,1}"/1
